simulink model "BUG2_V2"  (R2020a)
settings: Solver=VariableStepAuto  StartTime=0.0  StopTime=inf  RelTol=1e-3
libraries: robotlib x11
settings Model: Creator=root  LastModifiedBy=root

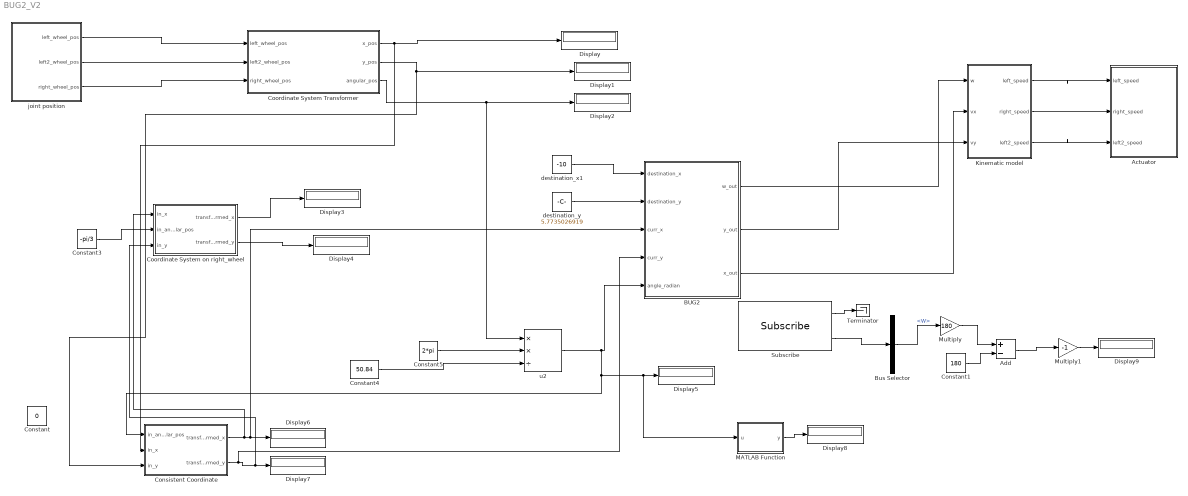
== system BUG2_V2 ==
  Actuator : Subsystem
  Add : Sum  Inputs=+-
  BUG2 : Subsystem
  Bus Selector : BusSelector  OutputSignals=Pose.Pose.Orientation.W
  Consistent Coordinate : Subsystem
  Constant : Constant  Value=0
  Constant1 : Constant  Value=180
  Constant3 : Constant  Value=-pi/3
  Constant4 : Constant  Value=50.84
  Constant5 : Constant  Value=2*pi
  Coordinate System Transformer : Subsystem
  Coordinate System on right_wheel : Subsystem
  Display{,1..9} (10 alike) : Display
  Kinematic model : Subsystem
  MATLAB Function : MATLAB Function  TreatAsAtomicUnit=on
  Multiply : Gain  Gain=180
  Multiply1 : Gain  Gain=-1
  Subscribe : robotlib/Subscribe  topicSource=Select from ROS network  topic=/odom  messageType=nav_msgs/Odometry  sampleTime=-1  messageQueueLength=1
  Terminator : Terminator
  destination_x1 : Constant  Value=-10
  destination_y : Constant  Value=5.7735026919
  joint position : Subsystem
  u2 : Product  Inputs=**/
  wires:
  Kinematic model/2(right_speed) -> Actuator/2(right_speed)
  Kinematic model/1(left_speed) -> Actuator/1(left_speed)
  Kinematic model/3(left2_speed) -> Actuator/3(left2_speed)
  BUG2/1(w_out) -> Kinematic model/1(w)
  joint position/1(left_wheel_pos) -> Coordinate System Transformer/1(left_wheel_pos)
  joint position/2(left2_wheel_pos) -> Coordinate System Transformer/2(left2_wheel_pos)
  Coordinate System Transformer/3(angular_pos) -> u2/1, Display2/1
  joint position/3(right_wheel_pos) -> Coordinate System Transformer/3(right_wheel_pos)
  Constant3/1 -> Coordinate System on right_wheel/2(in_angular_pos)
  Coordinate System on right_wheel/2(transformed_y) -> Display4/1
  Coordinate System on right_wheel/1(transformed_x) -> Display3/1
  destination_x1/1 -> BUG2/1(destination_x)
  destination_y/1 -> BUG2/2(destination_y)
  Constant4/1 -> u2/3
  Constant5/1 -> u2/2
  Consistent Coordinate/1(transformed_x) -> Coordinate System on right_wheel/1(in_x), BUG2/3(curr_x), Display6/1
  Consistent Coordinate/2(transformed_y) -> BUG2/4(curr_y), Coordinate System on right_wheel/3(in_y), Display7/1
  Coordinate System Transformer/1(x_pos) -> Consistent Coordinate/2(in_x), Display/1
  Coordinate System Transformer/2(y_pos) -> Consistent Coordinate/3(in_y), Display1/1
  BUG2/2(y_out) -> Kinematic model/3(vy)
  u2/1 -> Consistent Coordinate/1(in_angular_pos), MATLAB Function/1(u), Display5/1, BUG2/5(angle_radian)
  BUG2/3(x_out) -> Kinematic model/2(vx)
  MATLAB Function/1(y) -> Display8/1
  Subscribe/2 -> Bus Selector/1
  Bus Selector/1 -> Multiply/1  "<W>"
  Subscribe/1 -> Terminator/1
  Add/1 -> Multiply1/1
  Multiply/1 -> Add/1
  Constant1/1 -> Add/2
  Multiply1/1 -> Display9/1

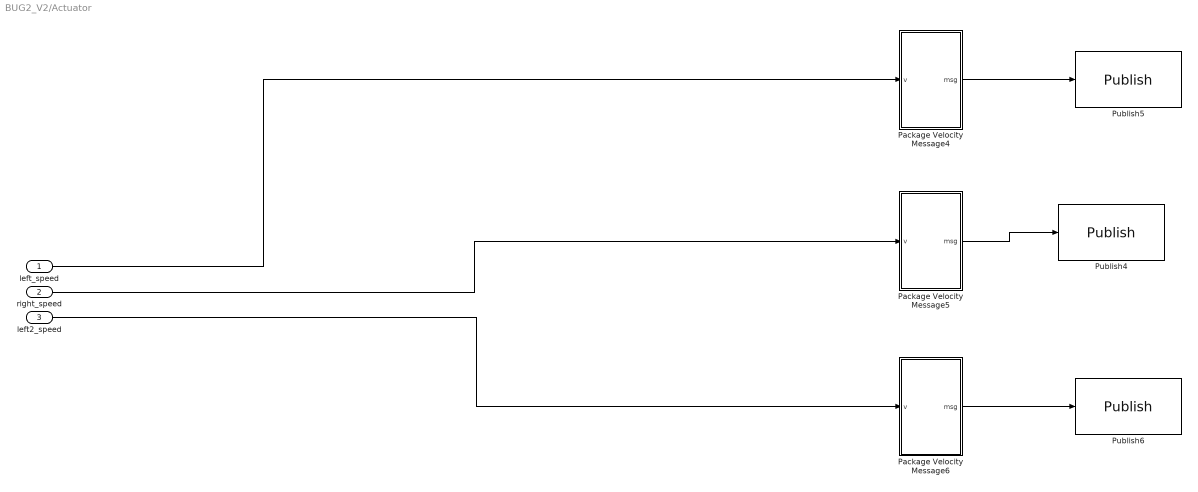
== system BUG2_V2/Actuator ==
  left_speed : Inport
  right_speed : Inport  Port=2
  left2_speed : Inport  Port=3
  Package Velocity Message4 : Subsystem
  Package Velocity Message5 : Subsystem
  Package Velocity Message6 : Subsystem
  Publish4 : robotlib/Publish  topicSource=Select from ROS network  topic=/robot/right_joint_velocity_controller/command  messageType=std_msgs/Float64  messageQueueLength=1
  Publish5 : robotlib/Publish  topicSource=Select from ROS network  topic=/robot/left_joint_velocity_controller/command  messageType=std_msgs/Float64  messageQueueLength=1
  Publish6 : robotlib/Publish  topicSource=Select from ROS network  topic=/robot/left2_joint_velocity_controller/command  messageType=std_msgs/Float64  messageQueueLength=1
  wires:
  left_speed/1 -> Package Velocity Message4/1(v)
  Package Velocity Message6/1(msg) -> Publish6/1
  right_speed/1 -> Package Velocity Message5/1(v)
  Package Velocity Message4/1(msg) -> Publish5/1
  Package Velocity Message5/1(msg) -> Publish4/1
  left2_speed/1 -> Package Velocity Message6/1(v)

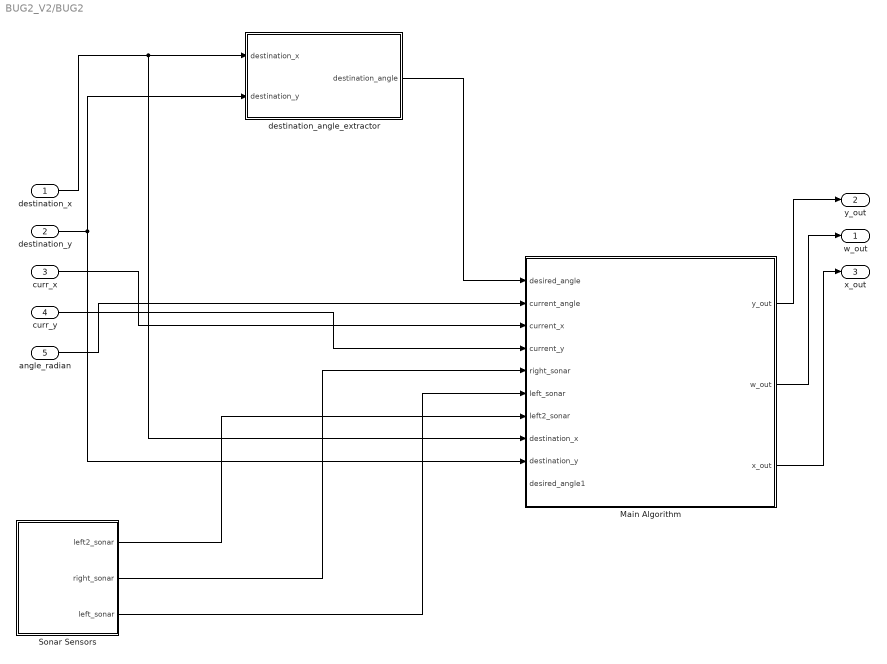
== system BUG2_V2/BUG2 ==
  destination_x : Inport
  destination_y : Inport  Port=2
  curr_x : Inport  Port=3
  curr_y : Inport  Port=4
  angle_radian : Inport  Port=5
  Main Algorithm : Stateflow chart  TreatAsAtomicUnit=on
  Sonar Sensors : Subsystem
  destination_angle_extractor : MATLAB Function  TreatAsAtomicUnit=on
  w_out : Outport
  y_out : Outport  Port=2
  x_out : Outport  Port=3
  wires:
  destination_x/1 -> Main Algorithm/8(destination_x), destination_angle_extractor/1(destination_x)
  angle_radian/1 -> Main Algorithm/2(current_angle)
  curr_y/1 -> Main Algorithm/4(current_y)
  curr_x/1 -> Main Algorithm/3(current_x)
  Main Algorithm/2(w_out) -> w_out/1
  destination_y/1 -> destination_angle_extractor/2(destination_y), Main Algorithm/9(destination_y)
  destination_angle_extractor/1(destination_angle) -> Main Algorithm/1(desired_angle)
  Main Algorithm/1(y_out) -> y_out/1
  Main Algorithm/3(x_out) -> x_out/1
  Sonar Sensors/1(left2_sonar) -> Main Algorithm/7(left2_sonar)
  Sonar Sensors/2(right_sonar) -> Main Algorithm/5(right_sonar)
  Sonar Sensors/3(left_sonar) -> Main Algorithm/6(left_sonar)

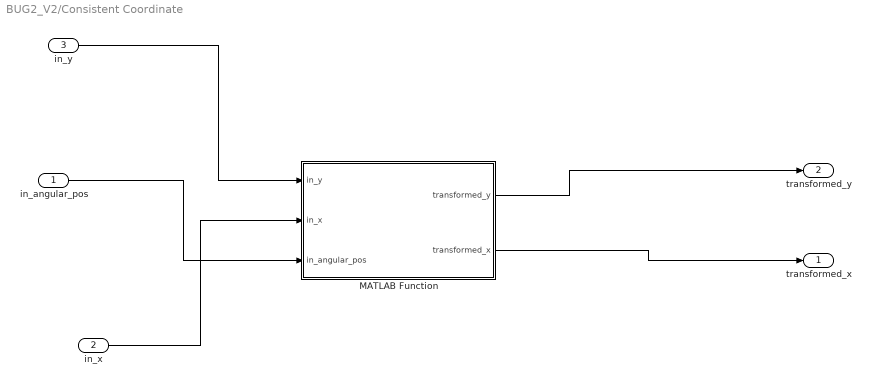
== system BUG2_V2/Consistent Coordinate ==
  in_angular_pos : Inport
  in_x : Inport  Port=2
  in_y : Inport  Port=3
  MATLAB Function : MATLAB Function  TreatAsAtomicUnit=on
  transformed_x : Outport
  transformed_y : Outport  Port=2
  wires:
  in_y/1 -> MATLAB Function/1(in_y)
  in_x/1 -> MATLAB Function/2(in_x)
  in_angular_pos/1 -> MATLAB Function/3(in_angular_pos)
  MATLAB Function/1(transformed_y) -> transformed_y/1
  MATLAB Function/2(transformed_x) -> transformed_x/1

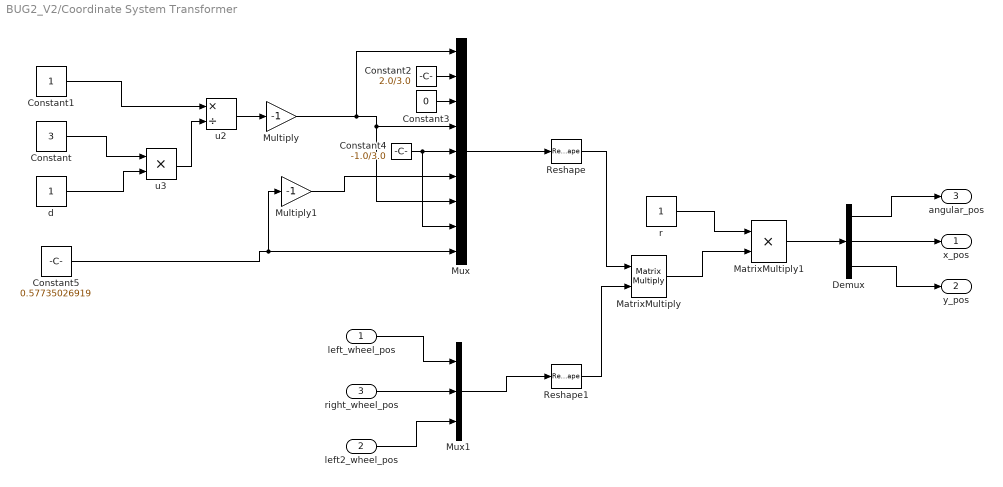
== system BUG2_V2/Coordinate System Transformer ==
  left_wheel_pos : Inport
  left2_wheel_pos : Inport  Port=2
  right_wheel_pos : Inport  Port=3
  Constant : Constant  Value=3
  Constant1 : Constant
  Constant2 : Constant  Value=2.0/3.0
  Constant3 : Constant  Value=0
  Constant4 : Constant  Value=-1.0/3.0
  Constant5 : Constant  Value=0.57735026919
  Demux : Demux  Outputs=3
  MatrixMultiply : Product  Multiplication=Matrix(*)
  MatrixMultiply1 : Product
  Multiply : Gain  Gain=-1
  Multiply1 : Gain  Gain=-1
  Mux : Mux  Inputs=9
  Mux1 : Mux  Inputs=3
  Reshape : Reshape  OutputDimensionality=Customize  OutputDimensions=[3,3]
  Reshape1 : Reshape  OutputDimensionality=Customize  OutputDimensions=[3,1]
  d : Constant
  r : Constant
  u2 : Product  Inputs=*/
  u3 : Product
  x_pos : Outport
  y_pos : Outport  Port=2
  angular_pos : Outport  Port=3
  wires:
  Constant1/1 -> u2/1
  d/1 -> u3/2
  Constant/1 -> u3/1
  u3/1 -> u2/2
  u2/1 -> Multiply/1
  Multiply/1 -> Mux/7, Mux/4, Mux/1
  Constant2/1 -> Mux/2
  Constant3/1 -> Mux/3
  Constant4/1 -> Mux/8, Mux/5
  Constant5/1 -> Multiply1/1, Mux/9
  Multiply1/1 -> Mux/6
  Mux/1 -> Reshape/1
  left_wheel_pos/1 -> Mux1/1
  right_wheel_pos/1 -> Mux1/2
  left2_wheel_pos/1 -> Mux1/3
  Mux1/1 -> Reshape1/1
  Reshape/1 -> MatrixMultiply/1
  Reshape1/1 -> MatrixMultiply/2
  r/1 -> MatrixMultiply1/1
  MatrixMultiply/1 -> MatrixMultiply1/2
  MatrixMultiply1/1 -> Demux/1
  Demux/1 -> angular_pos/1
  Demux/2 -> x_pos/1
  Demux/3 -> y_pos/1

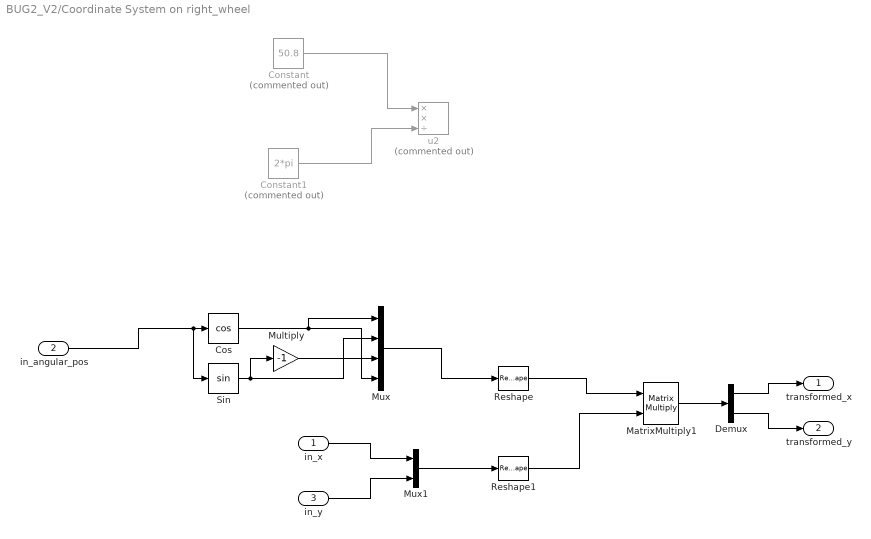
== system BUG2_V2/Coordinate System on right_wheel ==
  in_x : Inport
  in_angular_pos : Inport  Port=2
  in_y : Inport  Port=3
  Constant : Constant  Commented=on  Value=50.8
  Constant1 : Constant  Commented=on  Value=2*pi
  Cos : Trigonometry  Operator=cos
  Demux : Demux  Outputs=2
  MatrixMultiply1 : Product  Multiplication=Matrix(*)
  Multiply : Gain  Gain=-1
  Mux : Mux
  Mux1 : Mux  Inputs=2
  Reshape : Reshape  OutputDimensionality=Customize  OutputDimensions=[2,2]
  Reshape1 : Reshape  OutputDimensionality=Customize  OutputDimensions=[2,1]
  Sin : Trigonometry
  u2 : Product  Commented=on  Inputs=**/
  transformed_x : Outport
  transformed_y : Outport  Port=2
  wires:
  Constant1/1 -> u2/3
  Constant/1 -> u2/1
  Sin/1 -> Multiply/1, Mux/2
  Multiply/1 -> Mux/3
  Cos/1 -> Mux/4, Mux/1
  Mux/1 -> Reshape/1
  in_x/1 -> Mux1/1
  in_y/1 -> Mux1/2
  Mux1/1 -> Reshape1/1
  Reshape/1 -> MatrixMultiply1/1
  Reshape1/1 -> MatrixMultiply1/2
  MatrixMultiply1/1 -> Demux/1
  Demux/1 -> transformed_x/1
  Demux/2 -> transformed_y/1
  in_angular_pos/1 -> Sin/1, Cos/1

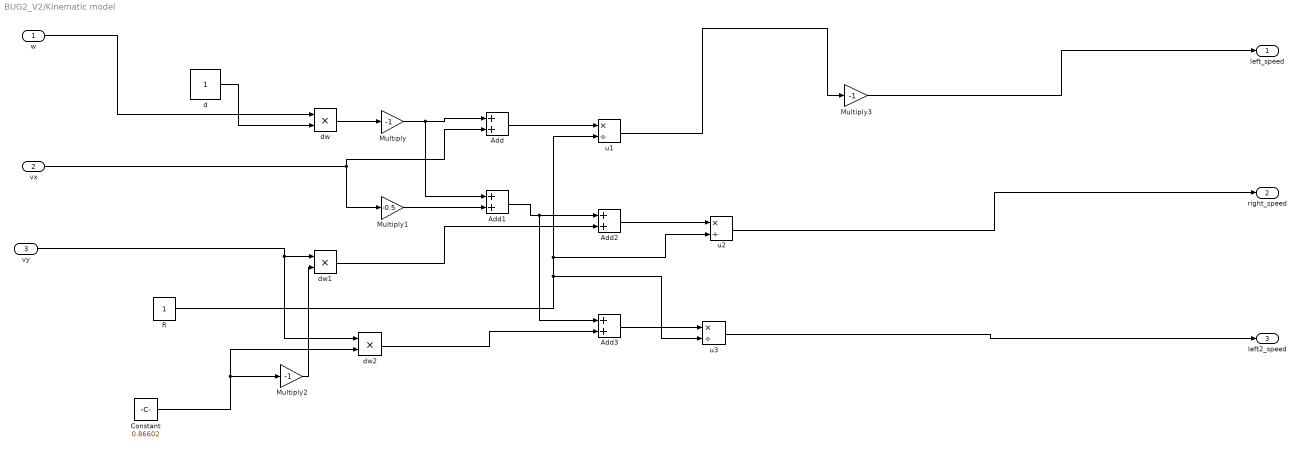
== system BUG2_V2/Kinematic model ==
  w : Inport
  vx : Inport  Port=2
  vy : Inport  Port=3
  Add{,1..3} (4 alike) : Sum
  Constant : Constant  Value=0.86602
  Multiply : Gain  Gain=-1
  Multiply1 : Gain  Gain=-0.5
  Multiply2 : Gain  Gain=-1
  Multiply3 : Gain  Gain=-1
  R : Constant
  d : Constant  VectorParams1D=off  SampleTime=-1
  dw : Product
  dw1 : Product
  dw2 : Product
  u1 : Product  Inputs=*/
  u2 : Product  Inputs=*/
  u3 : Product  Inputs=*/
  left_speed : Outport
  right_speed : Outport  Port=2
  left2_speed : Outport  Port=3
  wires:
  Multiply/1 -> Add1/1, Add/1
  Add/1 -> u1/1
  Multiply3/1 -> left_speed/1
  dw1/1 -> Add2/2
  w/1 -> dw/1
  Multiply2/1 -> dw1/2
  Add1/1 -> Add3/1, Add2/1
  Constant/1 -> dw2/2, Multiply2/1
  u3/1 -> left2_speed/1
  vy/1 -> dw2/1, dw1/1
  dw2/1 -> Add3/2
  d/1 -> dw/2
  u2/1 -> right_speed/1
  R/1 -> u3/2, u2/2, u1/2
  Add3/1 -> u3/1
  dw/1 -> Multiply/1
  vx/1 -> Add/2, Multiply1/1
  u1/1 -> Multiply3/1
  Add2/1 -> u2/1
  Multiply1/1 -> Add1/2

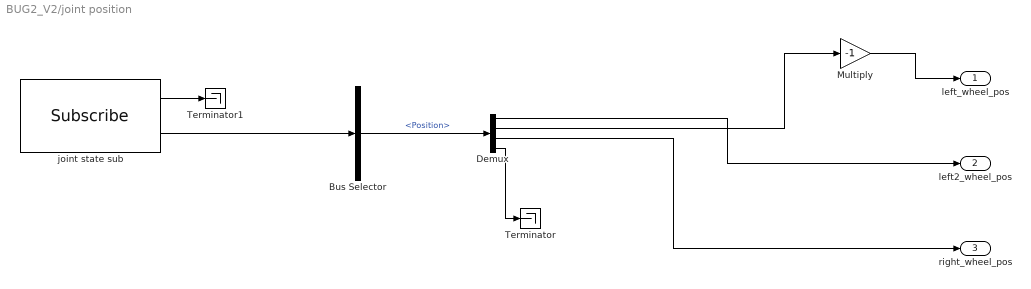
== system BUG2_V2/joint position ==
  Bus Selector : BusSelector  OutputSignals=Position
  Demux : Demux  Outputs=[1 1 1 -1]
  Multiply : Gain  Gain=-1
  Terminator : Terminator
  Terminator1 : Terminator
  joint state sub : robotlib/Subscribe  topicSource=Select from ROS network  topic=/robot/joint_states  messageType=sensor_msgs/JointState  sampleTime=-1  messageQueueLength=1
  left_wheel_pos : Outport
  left2_wheel_pos : Outport  Port=2
  right_wheel_pos : Outport  Port=3
  wires:
  joint state sub/2 -> Bus Selector/1
  Demux/2 -> Multiply/1
  Demux/3 -> right_wheel_pos/1
  Demux/1 -> left2_wheel_pos/1
  Bus Selector/1 -> Demux/1  "<Position>"
  Demux/4 -> Terminator/1
  Multiply/1 -> left_wheel_pos/1
  joint state sub/1 -> Terminator1/1

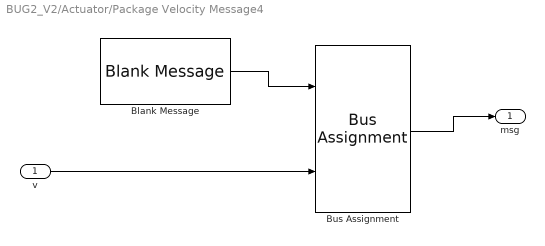
== system BUG2_V2/Actuator/Package Velocity Message4 ==
  v : Inport
  Blank Message : robotlib/Blank Message  messageClass=Message  entityType=std_msgs/Float64  messageType=std_msgs/Float64  SampleTime=inf
  Bus Assignment : BusAssignment  AssignedSignals=Data
  msg : Outport  VectorParamsAs1DForOutWhenUnconnected=off
  wires:
  Blank Message/1 -> Bus Assignment/1
  Bus Assignment/1 -> msg/1
  v/1 -> Bus Assignment/2

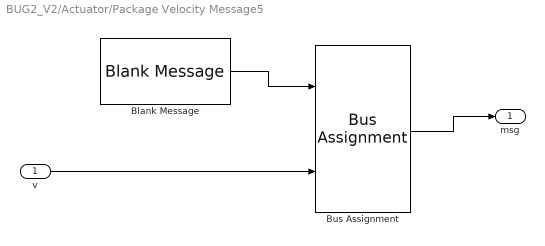
== system BUG2_V2/Actuator/Package Velocity Message5 ==
  v : Inport
  Blank Message : robotlib/Blank Message  messageClass=Message  entityType=std_msgs/Float64  messageType=std_msgs/Float64  SampleTime=inf
  Bus Assignment : BusAssignment  AssignedSignals=Data
  msg : Outport  VectorParamsAs1DForOutWhenUnconnected=off
  wires:
  Blank Message/1 -> Bus Assignment/1
  Bus Assignment/1 -> msg/1
  v/1 -> Bus Assignment/2

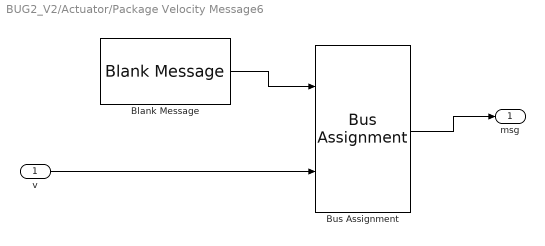
== system BUG2_V2/Actuator/Package Velocity Message6 ==
  v : Inport
  Blank Message : robotlib/Blank Message  messageClass=Message  entityType=std_msgs/Float64  messageType=std_msgs/Float64  SampleTime=inf
  Bus Assignment : BusAssignment  AssignedSignals=Data
  msg : Outport  VectorParamsAs1DForOutWhenUnconnected=off
  wires:
  Blank Message/1 -> Bus Assignment/1
  Bus Assignment/1 -> msg/1
  v/1 -> Bus Assignment/2

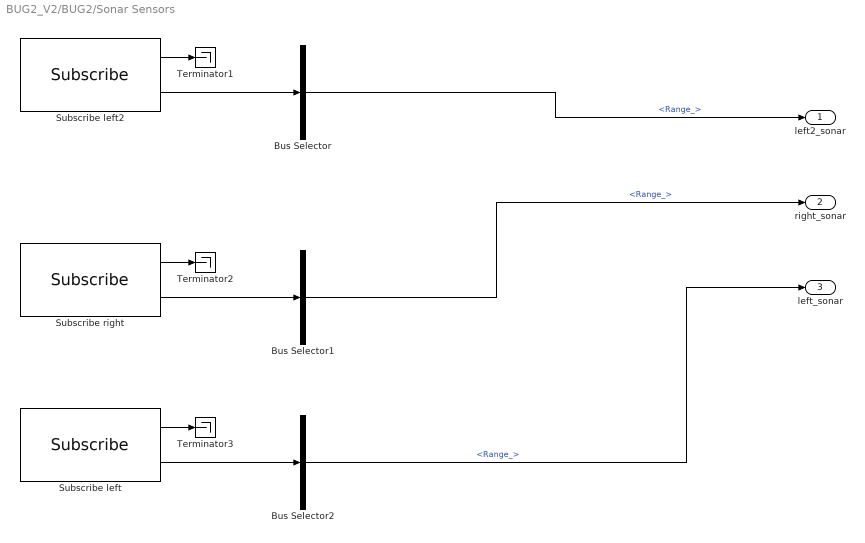
== system BUG2_V2/BUG2/Sonar Sensors ==
  Bus Selector : BusSelector  OutputSignals=Range_
  Bus Selector1 : BusSelector  OutputSignals=Range_
  Bus Selector2 : BusSelector  OutputSignals=Range_
  Subscribe left : robotlib/Subscribe  topicSource=Select from ROS network  topic=/sonar_sonar_link_3  messageType=sensor_msgs/Range  sampleTime=-1  messageQueueLength=1
  Subscribe left2 : robotlib/Subscribe  topicSource=Select from ROS network  topic=/sonar_sonar_link_1  messageType=sensor_msgs/Range  sampleTime=-1  messageQueueLength=1
  Subscribe right : robotlib/Subscribe  topicSource=Select from ROS network  topic=/sonar_sonar_link_2  messageType=sensor_msgs/Range  sampleTime=-1  messageQueueLength=1
  Terminator1 : Terminator
  Terminator2 : Terminator
  Terminator3 : Terminator
  left2_sonar : Outport
  right_sonar : Outport  Port=2
  left_sonar : Outport  Port=3
  wires:
  Bus Selector1/1 -> right_sonar/1  "<Range_>"
  Subscribe left/1 -> Terminator3/1
  Subscribe left/2 -> Bus Selector2/1
  Subscribe left2/1 -> Terminator1/1
  Subscribe right/1 -> Terminator2/1
  Bus Selector/1 -> left2_sonar/1  "<Range_>"
  Subscribe right/2 -> Bus Selector1/1
  Subscribe left2/2 -> Bus Selector/1
  Bus Selector2/1 -> left_sonar/1  "<Range_>"

== matlab function BUG2_V2/MATLAB Function ==
  data: u input; y output
function y = fcn(u)
y = mod((u*360)/(2*pi),360);
end

== matlab function BUG2_V2/Consistent Coordinate/MATLAB Function ==
  data: in_y input; transformed_y output; in_x input; in_angular_pos input; transformed_x output
function [transformed_y,transformed_x] = fcn(in_y, in_x, in_angular_pos)
    persistent cur_x;
    persistent cur_y;
    persistent last_in_y;
    persistent last_in_x;
    if(isempty(cur_x))
        cur_x = 0.0;
        cur_y = 0.0;
        last_in_x = 0.0;
        last_in_y = 0.0;
    end
    added_y = (in_y - last_in_y)*cos(-in_angular_pos) + (in_x - last_in_x)*sin(-in_angular_pos);
    added_x = -1*(in_y - last_in_y)*sin(-in_angular_pos) + (in_x - last_in_x)*cos(-in_angular_pos);
    cur_x = cur_x + added_x;
    cur_y = cur_y + added_y;
    last_in_x = in_x;
    last_in_y = in_y;
    transformed_y = cur_y;
    transformed_x = cur_x;
end

== matlab function BUG2_V2/BUG2/destination_angle_extractor ==
  data: destination_x input; destination_angle output; destination_y input
function destination_angle = fcn(destination_x, destination_y)
 raw_angle = atan(destination_x/destination_y);
 destination_angle = raw_angle;
 if raw_angle >= 0 && (destination_x <0 || destination_y < 0)
  destination_angle = raw_angle + pi;
 elseif raw_angle < 0 && (destination_y < 0 || destination_x > 0)
  destination_angle = raw_angle + pi;
 end
 destination_angle = mod(pi + destination_angle, 2*pi);
 if(abs(destination_angle - 2*pi) < abs(destination_angle))
     destination_angle = abs(destination_angle - 2*pi);
 end
 if(abs(destination_angle + 2*pi) < abs(destination_angle))
     destination_angle = abs(destination_angle + 2*pi);
 end    
     
end

== stateflow chart BUG2_V2/BUG2/Main Algorithm ==
  state INIT
    rot_pos_margin = 0.01;
    rot_vel_gain = 2;
    lin_vel_gain = 4;
    w_out = 0;
    x_out = 0;
    y_out = 0;
    sonar_margin = 0.7;
    max_sonar = 1.4;
  state INITIAL_ANGLE_CHANGER
    entry:
    w_out = rot_vel_gain*(desired_angle - current_angle)/abs(desired_angle - current_angle);
    x_out = 0;
    y_out = 0;
  state MOVE_TOWARD
    entry:
    w_out = 0;
    y_out = -1*lin_vel_gain;
    x_out = 0;
  state OBSTACLE_AVOID
    entry:
    w_out = 0;
    y_out = 0;
    x_out = 1*lin_vel_gain;
  state MOVE_FAR
    entry:
    w_out = rot_vel_gain * (-1);
    y_out = 0;
    x_out = 0;
    move_around = 1;
  state INIT_MOVE_NEAR
    entry:
    y_out = -0.7*lin_vel_gain;
    x_out = 0;
    w_out = 0;
    move_around = 1;
  state MOVE_NEAR
    entry:
    w_out = rot_vel_gain * (1);
    y_out = 0;
    x_out = 0;
    move_around = 1;
  OBSTACLE_AVOID -> INITIAL_ANGLE_CHANGER [order 1] : [move_around == 1 && (abs(current_grad-destination_grad)< 0.01)]
  (default) -> INIT
  INIT -> INITIAL_ANGLE_CHANGER
  INITIAL_ANGLE_CHANGER -> MOVE_TOWARD : [mod(abs(desired_angle-current_angle),2*pi) < rot_pos_margin ]
  MOVE_TOWARD -> OBSTACLE_AVOID : [left_sonar < sonar_margin]{last_left_sonar = left_sonar, move_around = 0;destination_grad = destination_y/destination_x;
      | current_grad = current_y/current_x;}
  MOVE_NEAR -> OBSTACLE_AVOID [order 1] : [ left_sonar > last_left_sonar || left_sonar < sonar_margin || left_sonar == max_sonar]
  OBSTACLE_AVOID -> OBSTACLE_AVOID [order 4] : {destination_grad = destination_y/destination_x;
      | current_grad = current_y/current_x;}
  OBSTACLE_AVOID -> INIT_MOVE_NEAR [order 2] : [left_sonar - sonar_margin > 0.1*sonar_margin ]{last_left_sonar = left_sonar}
  OBSTACLE_AVOID -> MOVE_FAR [order 3] : [ 0.2*sonar_margin < sonar_margin - left_sonar ]{last_left_sonar = left_sonar}
  MOVE_FAR -> OBSTACLE_AVOID [order 1] : [left_sonar < last_left_sonar || left_sonar > 0.8*sonar_margin]
  INIT_MOVE_NEAR -> MOVE_NEAR : [after(400,msec)]
  MOVE_FAR -> MOVE_FAR [order 2] : {last_left_sonar = left_sonar}
  MOVE_NEAR -> MOVE_NEAR [order 2] : {last_left_sonar = left_sonar}
  data: y_out output; desired_angle input; current_angle input; rot_vel_gain local; rot_pos_margin local; w_out output; x_out output; current_x input; current_y input; right_sonar input; left_sonar input; left2_sonar input; lin_vel_gain local; sonar_margin local; last_left_sonar local; max_sonar local; destination_x input; destination_y input; current_grad local; destination_grad local; move_around local; desired_angle1 input
